simulink model "Viento_coordenadas"  (R2020a)
settings: Solver=VariableStepAuto  StartTime=0.0  StopTime=20  RelTol=1e-3
values from neighbouring files (symbols this model uses):
  Areavector = [0.293;0.022;0.022]    [Iteradorcompleto.m]    (also in Parametros_iniciales.m)
  body_rate_0 = [0;0;0]    [Iteradorcompleto.m]    (also in Parametros_iniciales.m)
  cd = 0.2    [Iteradorcompleto.m]    (also in Parametros_iniciales.m)
  Euler_0 = [0;0;0]    [Iteradorcompleto.m]    (also in Parametros_iniciales.m)
  g = [0;0;-3.66]    [Iteradorcompleto.m]    (also in Parametros_iniciales.m)
  I = [[0.01739,0,0];[0,0.01739,0];[0,0,0.0225]]    [Iteradorcompleto.m]    (also in Parametros_iniciales.m)
  m = T_V1toI*T_V2toV1*T_BtoV2    [Creacion_animacion.m]    (also in Iteradorcompleto.m = 2; Parametros_iniciales.m = 2)
  rho = 0.0195    [Iteradorcompleto.m]    (also in Parametros_iniciales.m)
  ts = 0.01    [Iteradorcompleto.m]    (also in Parametros_iniciales.m)
  vwind = real(-C*(log(1-probabilidad))^(1/K))    [DistribucionWeibul.m]    (also in Iteradorcompleto.m)
  XYZ_0 = [0;0;0]    [Iteradorcompleto.m]    (also in Parametros_iniciales.m = [0;0;5])
libraries: simulink x51, vrlib x2, aerolibutil x1
(part 1 of 4)
settings Model: NumberOfSteps=10  Creator=blaze8871  LastModifiedBy=Portatil
settings DataIOCC: SaveTime=off

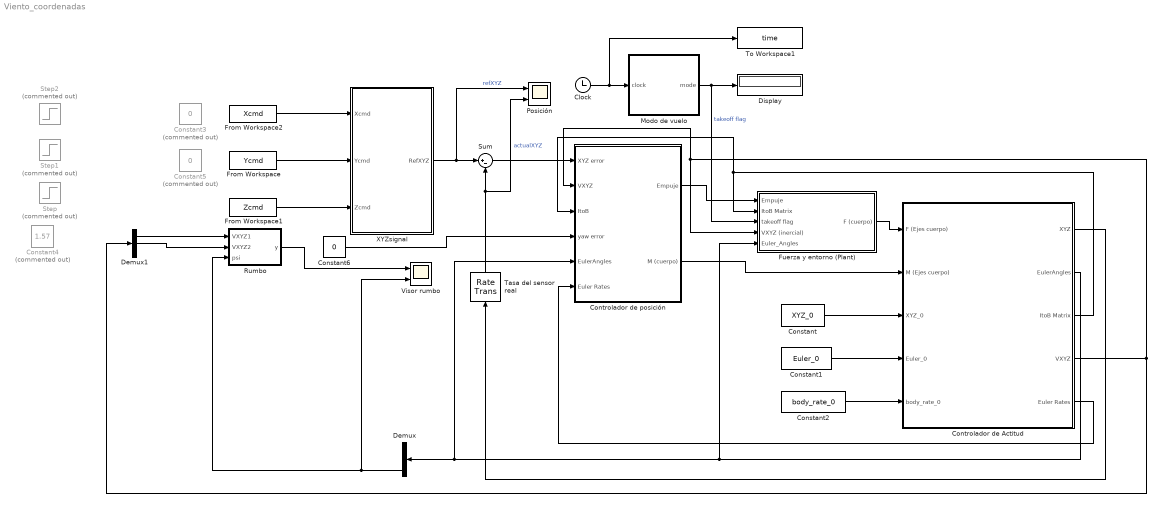
== system Viento_coordenadas ==
  Clock : Clock
  Constant : Constant  Value=XYZ_0  SampleTime=-1
  Constant1 : Constant  Value=Euler_0  SampleTime=-1
  Constant2 : Constant  Value=body_rate_0  SampleTime=-1
  Constant3 : Constant  Commented=on  Value=0
  Constant4 : Constant  Commented=on  Value=1.57
  Constant5 : Constant  Commented=on  Value=0
  Constant6 : Constant  Value=0
  Controlador de Actitud : Subsystem
  Controlador de posición : Subsystem
  Demux : Demux  Outputs=3
  Demux1 : Demux  Outputs=3
  Display : Display
  From Workspace : FromWorkspace  VariableName=Ycmd  SampleTime=ts
  From Workspace1 : FromWorkspace  VariableName=Zcmd  SampleTime=ts
  From Workspace2 : FromWorkspace  VariableName=Xcmd  SampleTime=ts
  Fuerza y entorno (Plant) : Subsystem
  Modo de vuelo : MATLAB Function  TreatAsAtomicUnit=on
  Posición : Scope  NumInputPorts=2
  Rumbo : MATLAB Function  TreatAsAtomicUnit=on
  Step : Step  Commented=on  Time=0  SampleTime=ts
  Step1 : Step  Commented=on  Time=2  SampleTime=ts
  Step2 : Step  Commented=on  Time=3  SampleTime=ts
  Sum : Sum  Inputs=|+-
  Tasa del sensor real : RateTransition  OutPortSampleTime=ts
  To Workspace1 : ToWorkspace  VariableName=time  SampleTime=ts
  Visor rumbo : Scope  NumInputPorts=2
  XYZsignal : MATLAB Function  TreatAsAtomicUnit=on
  wires:
  Constant/1 -> Controlador de Actitud/3(XYZ_0)
  Constant1/1 -> Controlador de Actitud/4(Euler_0)
  Constant2/1 -> Controlador de Actitud/5(body_rate_0)
  XYZsignal/1(RefXYZ) -> Sum/1, Posición/1  "refXYZ"
  Controlador de Actitud/1(XYZ) -> Tasa del sensor real/1
  Clock/1 -> To Workspace1/1, Modo de vuelo/1(clock)
  Modo de vuelo/1(mode) -> Fuerza y entorno (Plant)/3(takeoff flag), Display/1  "takeoff flag"
  Fuerza y entorno (Plant)/1(F (cuerpo)) -> Controlador de Actitud/1(F (Ejes cuerpo))
  Controlador de Actitud/2(EulerAngles) -> Fuerza y entorno (Plant)/5(Euler_Angles), Demux/1, Controlador de posición/5(EulerAngles)
  Sum/1 -> Controlador de posición/1(XYZ error)
  Controlador de posición/2(M (cuerpo)) -> Controlador de Actitud/2(M (Ejes cuerpo))
  Controlador de posición/1(Empuje) -> Fuerza y entorno (Plant)/1(Empuje)
  Tasa del sensor real/1 -> Posición/2, Sum/2  "actualXYZ"
  Controlador de Actitud/5(Euler Rates) -> Controlador de posición/6(Euler Rates)
  Controlador de Actitud/3(ItoB Matrix) -> Controlador de posición/3(ItoB), Fuerza y entorno (Plant)/2(ItoB Matrix)
  Demux/3 -> Rumbo/3(psi), Visor rumbo/2
  Controlador de Actitud/4(VXYZ) -> Demux1/1, Controlador de posición/2(VXYZ), Fuerza y entorno (Plant)/4(VXYZ (inercial))
  Demux1/1 -> Rumbo/1(VXYZ1)
  Demux1/2 -> Rumbo/2(VXYZ2)
  Rumbo/1(y) -> Visor rumbo/1
  From Workspace2/1 -> XYZsignal/1(Xcmd)
  From Workspace/1 -> XYZsignal/2(Ycmd)
  From Workspace1/1 -> XYZsignal/3(Zcmd)
  Constant6/1 -> Controlador de posición/4(yaw error)

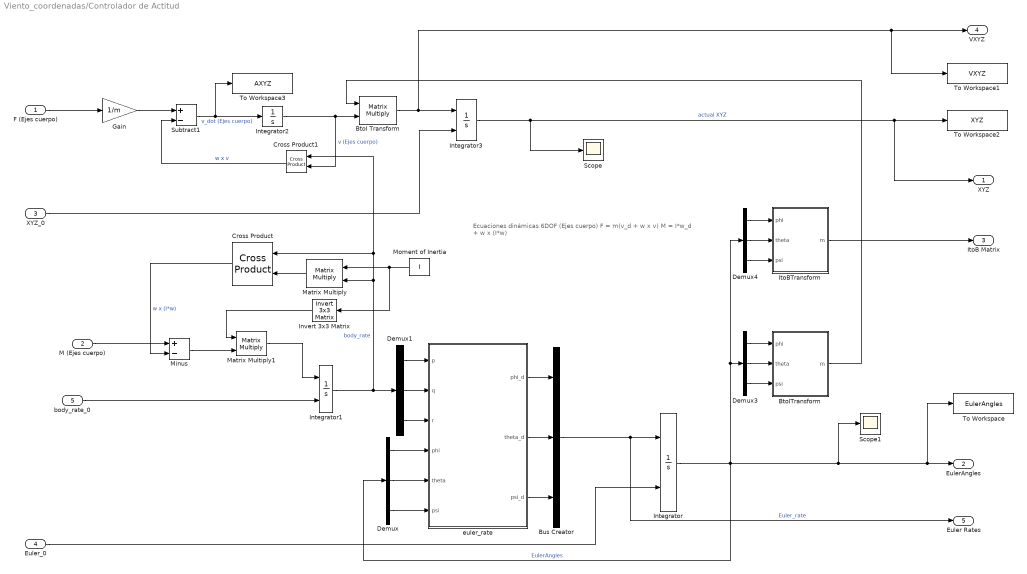
== system Viento_coordenadas/Controlador de Actitud ==
  note: Ecuaciones dinámicas 6DOF
      | (Ejes cuerpo)
      |
      | F = m(v_d + w x v)
      | M = I*w_d + w x (I*w)
  F (Ejes cuerpo) : Inport
  M (Ejes cuerpo) : Inport  Port=2
  XYZ_0 : Inport  Port=3
  Euler_0 : Inport  Port=4
  body_rate_0 : Inport  Port=5
  BtoI Transform : Product  Multiplication=Matrix(*)
  BtoITransform : MATLAB Function  TreatAsAtomicUnit=on
  Bus Creator : BusCreator  Inputs=3
  Cross Product : vrlib/Utilities/Cross Product
  Cross Product1 : vrlib/Utilities/Cross Product
  Demux{,1,3..4} (4 alike) : Demux  Outputs=3
  Gain : Gain  Gain=1/m
  Integrator : Integrator  InitialConditionSource=external  ContinuousStateAttributes='EulerAngle'
  Integrator1 : Integrator  InitialConditionSource=external  ContinuousStateAttributes='EulerAngle'
  Integrator2 : Integrator
  Integrator3 : Integrator  InitialConditionSource=external
  Invert 3x3 Matrix : aerolibutil/Invert  3x3 Matrix
  ItoBTransform : MATLAB Function  TreatAsAtomicUnit=on
  Matrix Multiply : Product  Multiplication=Matrix(*)
  Matrix Multiply1 : Product  Multiplication=Matrix(*)
  Minus : Sum  Inputs=+-
  Moment of Inertia : Constant  Value=I
  Scope : Scope
  Scope1 : Scope
  Subtract1 : Sum  Inputs=+-
  To Workspace : ToWorkspace  VariableName=EulerAngles  SampleTime=ts
  To Workspace1 : ToWorkspace  VariableName=VXYZ  SampleTime=ts
  To Workspace2 : ToWorkspace  VariableName=XYZ  SampleTime=ts
  To Workspace3 : ToWorkspace  VariableName=AXYZ  SampleTime=ts
  euler_rate : MATLAB Function  TreatAsAtomicUnit=on
  XYZ : Outport
  EulerAngles : Outport  Port=2
  ItoB Matrix : Outport  Port=3
  VXYZ : Outport  Port=4
  Euler Rates : Outport  Port=5
  wires:
  F (Ejes cuerpo)/1 -> Gain/1
  Demux4/2 -> ItoBTransform/2(theta)
  euler_rate/1(phi_d) -> Bus Creator/1
  BtoITransform/1(m) -> BtoI Transform/1
  Bus Creator/1 -> Euler Rates/1, Integrator/1  "Euler_rate"
  Matrix Multiply/1 -> Cross Product/2
  Moment of Inertia/1 -> Invert 3x3 Matrix/1, Matrix Multiply/1
  Demux3/2 -> BtoITransform/2(theta)
  Demux/2 -> euler_rate/5(theta)
  Demux4/1 -> ItoBTransform/1(phi)
  Subtract1/1 -> To Workspace3/1, Integrator2/1  "v_dot (Ejes cuerpo)"
  Cross Product1/1 -> Subtract1/2  "w x v"
  Demux1/1 -> euler_rate/1(p)
  Demux/3 -> euler_rate/6(psi)
  euler_rate/2(theta_d) -> Bus Creator/2
  Euler_0/1 -> Integrator/2
  Integrator3/1 -> XYZ/1, To Workspace2/1, Scope/1  "actual XYZ"
  Cross Product/1 -> Minus/2  "w x (I*w)"
  M (Ejes cuerpo)/1 -> Minus/1
  body_rate_0/1 -> Integrator1/2
  Demux3/3 -> BtoITransform/3(psi)
  euler_rate/3(psi_d) -> Bus Creator/3
  Demux4/3 -> ItoBTransform/3(psi)
  Gain/1 -> Subtract1/1
  Demux3/1 -> BtoITransform/1(phi)
  Demux1/3 -> euler_rate/3(r)
  XYZ_0/1 -> Integrator3/2
  Integrator/1 -> Demux/1, Scope1/1, To Workspace/1, EulerAngles/1, Demux4/1, Demux3/1  "EulerAngles"
  Demux/1 -> euler_rate/4(phi)
  Integrator2/1 -> BtoI Transform/2, Cross Product1/2  "v (Ejes cuerpo)"
  Integrator1/1 -> Cross Product1/1, Cross Product/1, Matrix Multiply/2, Demux1/1  "body_rate"
  Demux1/2 -> euler_rate/2(q)
  ItoBTransform/1(m) -> ItoB Matrix/1
  BtoI Transform/1 -> To Workspace1/1, VXYZ/1, Integrator3/1
  Minus/1 -> Matrix Multiply1/2
  Matrix Multiply1/1 -> Integrator1/1
  Invert 3x3 Matrix/1 -> Matrix Multiply1/1

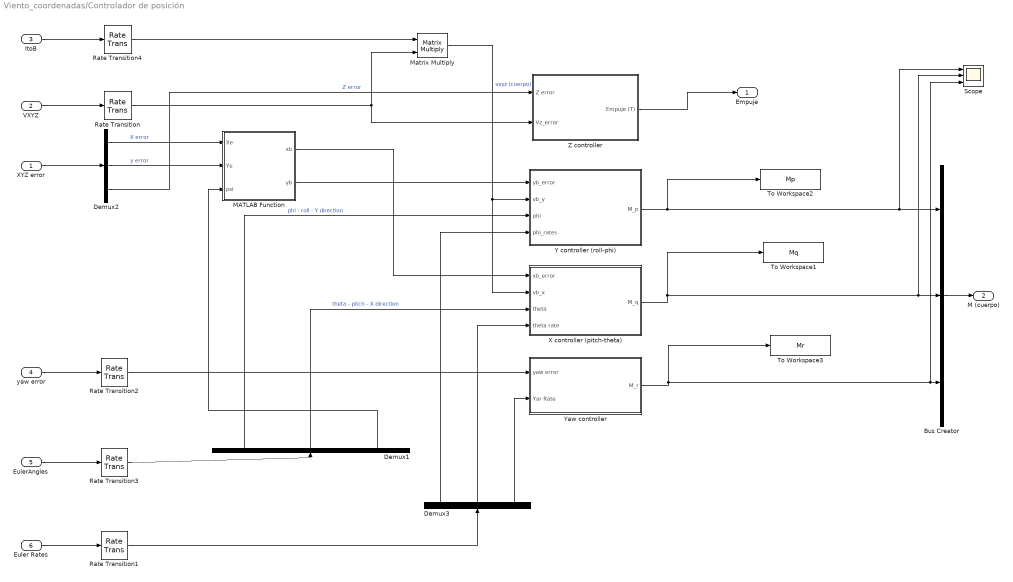
== system Viento_coordenadas/Controlador de posición ==
  XYZ error : Inport
  VXYZ : Inport  Port=2
  ItoB : Inport  Port=3
  yaw error : Inport  Port=4
  EulerAngles : Inport  Port=5
  Euler Rates : Inport  Port=6
  Bus Creator : BusCreator  Inputs=3
  Demux1 : Demux  Outputs=3
  Demux2 : Demux  Outputs=3
  Demux3 : Demux  Outputs=3
  MATLAB Function : MATLAB Function  TreatAsAtomicUnit=on
  Matrix Multiply : Product  Multiplication=Matrix(*)
  Rate Transition{,1..4} (5 alike) : RateTransition  OutPortSampleTime=ts
  Scope : Scope  NumInputPorts=3
  To Workspace1 : ToWorkspace  VariableName=Mq  SampleTime=0.01
  To Workspace2 : ToWorkspace  VariableName=Mp  SampleTime=0.01
  To Workspace3 : ToWorkspace  VariableName=Mr  SampleTime=0.01
  X controller (pitch-theta) : Subsystem
  Y controller (roll-phi) : Subsystem
  "Yaw controller " : Subsystem
  Z controller : Subsystem
  Empuje : Outport
  M (cuerpo) : Outport  Port=2
  wires:
  Bus Creator/1 -> M (cuerpo)/1
  VXYZ/1 -> Rate Transition/1
  "Yaw controller "/1(M_r) -> To Workspace3/1, Scope/3, Bus Creator/3
  Demux2/3 -> Z controller/1(Z error)  "Z error"
  EulerAngles/1 -> Rate Transition3/1
  Y controller (roll-phi)/1(M_p) -> Scope/1, Bus Creator/1, To Workspace2/1
  Demux1/3 -> MATLAB Function/3(psi)
  Z controller/1(Empuje (T)) -> Empuje/1
  Demux2/2 -> MATLAB Function/2(Ye)  "y error"
  yaw error/1 -> Rate Transition2/1
  Demux2/1 -> MATLAB Function/1(Xe)  "X error"
  X controller (pitch-theta)/1(M_q) -> To Workspace1/1, Scope/2, Bus Creator/2
  MATLAB Function/1(xb) -> X controller (pitch-theta)/1("xb_error ")
  MATLAB Function/2(yb) -> Y controller (roll-phi)/1("yb_error ")
  ItoB/1 -> Rate Transition4/1
  Matrix Multiply/1 -> X controller (pitch-theta)/2(vb_x), Y controller (roll-phi)/2(vb_y)  "vxyz (cuerpo)"
  Rate Transition/1 -> Z controller/2(Vz_error), Matrix Multiply/2
  XYZ error/1 -> Demux2/1
  Rate Transition2/1 -> "Yaw controller "/1(yaw error)
  Rate Transition3/1 -> Demux1/1
  Rate Transition4/1 -> Matrix Multiply/1
  Euler Rates/1 -> Rate Transition1/1
  Rate Transition1/1 -> Demux3/1
  Demux3/3 -> "Yaw controller "/2(Yar Rate)
  Demux3/2 -> X controller (pitch-theta)/4(theta rate)
  Demux1/2 -> X controller (pitch-theta)/3(theta)  "theta - pitch - X direction"
  Demux1/1 -> Y controller (roll-phi)/3(phi)  "phi - roll - Y direction"
  Demux3/1 -> Y controller (roll-phi)/4(phi_rates)

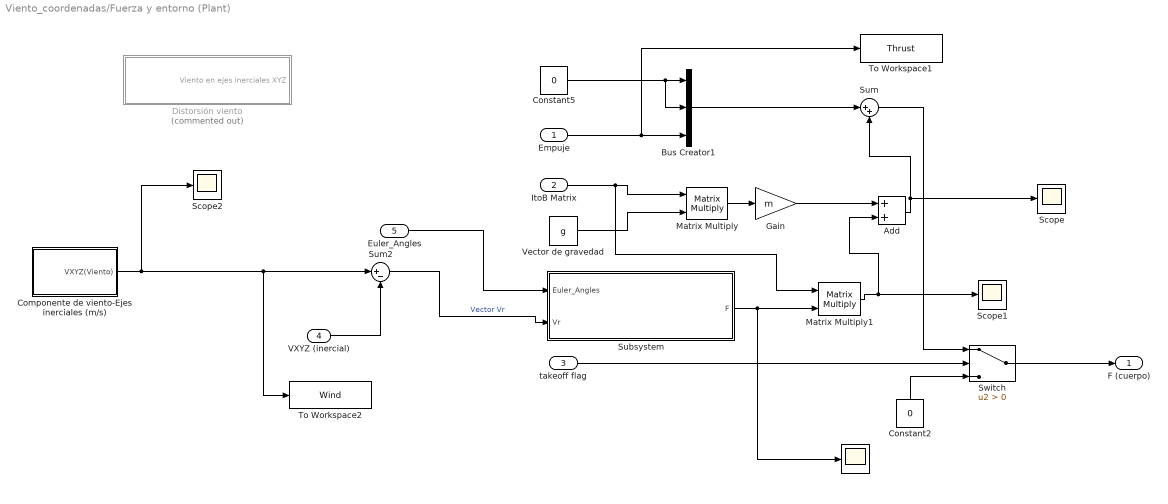
== system Viento_coordenadas/Fuerza y entorno (Plant) ==
  Empuje : Inport
  ItoB Matrix : Inport  Port=2
  takeoff flag : Inport  Port=3
  VXYZ (inercial) : Inport  Port=4
  Euler_Angles : Inport  Port=5
  " " : Scope
  Add : Sum
  Bus Creator1 : BusCreator  Inputs=3
  Componente de viento-Ejes inerciales (m/s) : Subsystem
  Constant2 : Constant  Value=0  SampleTime=-1
  Constant5 : Constant  Value=0  SampleTime=-1
  Distorsión viento : Subsystem  Commented=on
  Gain : Gain  Gain=m
  Matrix Multiply : Product  Multiplication=Matrix(*)
  Matrix Multiply1 : Product  Multiplication=Matrix(*)
  Scope : Scope
  Scope1 : Scope
  Scope2 : Scope
  Subsystem : Subsystem
  Sum : Sum  Inputs=|++
  Sum2 : Sum  Inputs=|+-
  Switch : Switch  Criteria=u2 > Threshold
  To Workspace1 : ToWorkspace  VariableName=Thrust  SampleTime=0.01
  To Workspace2 : ToWorkspace  VariableName=Wind  SampleTime=0.01
  Vector de gravedad : Constant  Value=g  SampleTime=-1
  F (cuerpo) : Outport
  wires:
  Empuje/1 -> To Workspace1/1, Bus Creator1/3
  Bus Creator1/1 -> Sum/1
  ItoB Matrix/1 -> Matrix Multiply1/1, Matrix Multiply/1
  Constant5/1 -> Bus Creator1/2, Bus Creator1/1
  takeoff flag/1 -> Switch/2
  Constant2/1 -> Switch/3
  Matrix Multiply/1 -> Gain/1
  Sum/1 -> Switch/1
  Switch/1 -> F (cuerpo)/1
  Vector de gravedad/1 -> Matrix Multiply/2
  VXYZ (inercial)/1 -> Sum2/2
  Sum2/1 -> Subsystem/2(Vr)  "Vector Vr"
  Euler_Angles/1 -> Subsystem/1(Euler_Angles)
  Subsystem/1(F) -> " "/1, Matrix Multiply1/2
  Add/1 -> Scope/1, Sum/2
  Gain/1 -> Add/1
  Matrix Multiply1/1 -> Add/2, Scope1/1
  Componente de viento-Ejes inerciales (m/s)/1(VXYZ(Viento)) -> Scope2/1, To Workspace2/1, Sum2/1
